simulink model "vechicle_circular_traversing"  (R2018b)
settings: Solver=FixedStepDiscrete  StartTime=0.0  StopTime=TFinal  FixedStep=Ts  RelTol=1e-3
values from neighbouring files (symbols this model uses):
  cx = 2    [Test_EKF_circular_trajectory.m]
  cy = 2    [Test_EKF_circular_trajectory.m]
  muWx = 0    [Test_EKF_circular_trajectory.m]
  muWy = 0    [Test_EKF_circular_trajectory.m]
  P0 = [1;1]    [Test_EKF_circular_trajectory.m]
  sigB = 1e-1    (= 0.1)    [Test_EKF_circular_trajectory.m]
  sigR = 1e-1    (= 0.1)    [Test_EKF_circular_trajectory.m]
  sigWx = 1e-7    (= 1e-07)    [Test_EKF_circular_trajectory.m]
  sigWy = 1e-7    (= 1e-07)    [Test_EKF_circular_trajectory.m]
  Ts = 0.01    [KF_Pendulum_parameter.m]    (also in Test_EKF_circular_trajectory.m)
  V0 = [-0.25;0.25]    [Test_EKF_circular_trajectory.m]
  wx = 0    [Test_EKF_circular_trajectory.m]
  wy = 0    [Test_EKF_circular_trajectory.m]
  Z = 2    [Test_EKF_circular_trajectory.m]
undefined symbols (not defined in the file or in its folder): randraw
settings Model: Creator=chpark  LastModifiedBy=chpark

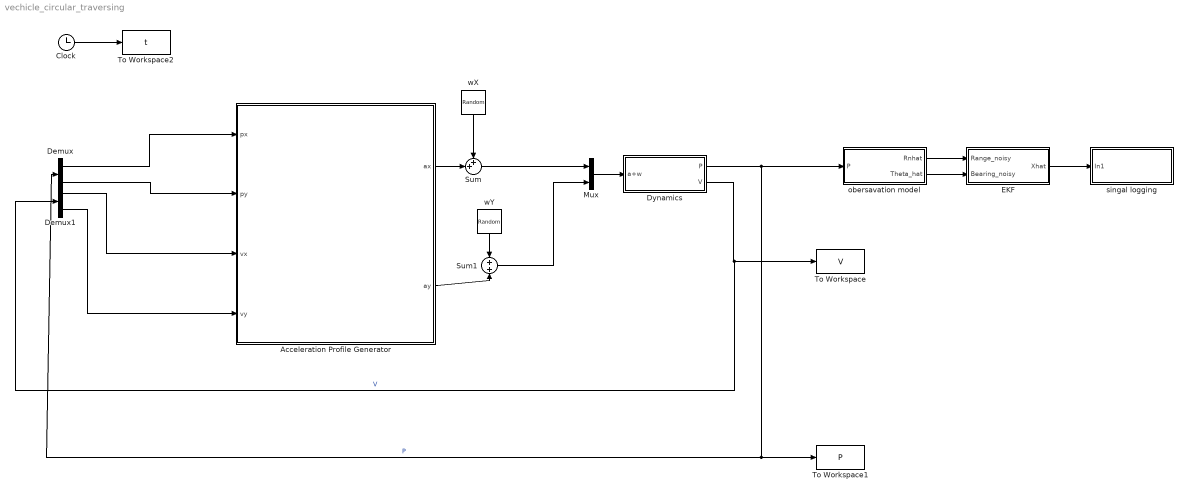
== system vechicle_circular_traversing ==
  Acceleration Profile Generator : Subsystem
  Clock : Clock
  Demux : Demux  Outputs=2
  Demux1 : Demux  Outputs=2
  Dynamics : Subsystem
  EKF : Subsystem
  Mux : Mux  Inputs=2
  Sum : Sum  Inputs=++|
  Sum1 : Sum
  To Workspace : ToWorkspace  VariableName=V  SampleTime=-1
  To Workspace1 : ToWorkspace  VariableName=P  SampleTime=-1
  To Workspace2 : ToWorkspace  VariableName=t  SampleTime=-1
  obersavation model : Subsystem
  singal logging : Subsystem
  wX : RandomNumber  Mean=muWx  Variance=sigWx  Seed=2^wx  SampleTime=Ts
  wY : RandomNumber  Mean=muWy  Variance=sigWy  Seed=2^wy  SampleTime=Ts
  wires:
  Acceleration Profile Generator/1(ax) -> Sum/2
  wX/1 -> Sum/1
  wY/1 -> Sum1/1
  Acceleration Profile Generator/2(ay) -> Sum1/2
  Sum1/1 -> Mux/2
  Sum/1 -> Mux/1
  Mux/1 -> Dynamics/1(a+w)
  Dynamics/1(P) -> obersavation model/1(P), To Workspace1/1, Demux/1  "P"
  obersavation model/1(Rnhat) -> EKF/1(Range_noisy)
  obersavation model/2(Theta_hat) -> EKF/2(Bearing_noisy)
  EKF/1(Xhat) -> singal logging/1(In1)
  Demux/1 -> Acceleration Profile Generator/1(px)
  Demux/2 -> Acceleration Profile Generator/2(py)
  Demux1/1 -> Acceleration Profile Generator/3(vx)
  Demux1/2 -> Acceleration Profile Generator/4(vy)
  Dynamics/2(V) -> Demux1/1, To Workspace/1  "V"
  Clock/1 -> To Workspace2/1

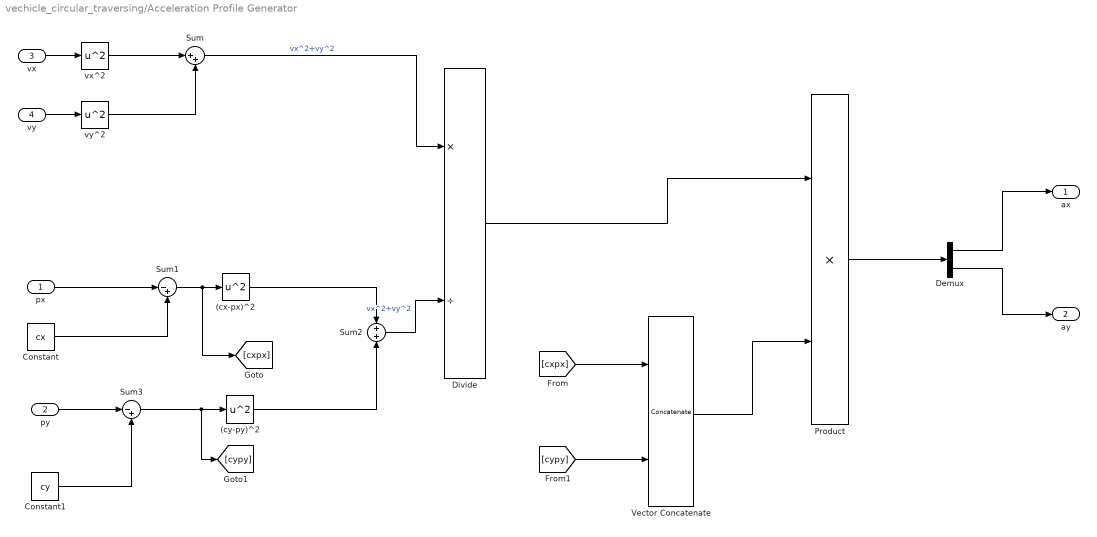
== system vechicle_circular_traversing/Acceleration Profile Generator ==
  px : Inport
  py : Inport  Port=2
  vx : Inport  Port=3
  vy : Inport  Port=4
  (cx-px)^2 : Math  Operator=square  SaturateOnIntegerOverflow=on
  (cy-py)^2 : Math  Operator=square  SaturateOnIntegerOverflow=on
  Constant : Constant  Value=cx
  Constant1 : Constant  Value=cy
  Demux : Demux  Outputs=2
  Divide : Product  Inputs=*/
  Product : Product
  Sum : Sum  Inputs=|++
  Sum1 : Sum  Inputs=|-+
  Sum2 : Sum
  Sum3 : Sum  Inputs=|-+
  Vector Concatenate : Concatenate
  vx^2 : Math  Operator=square  SaturateOnIntegerOverflow=on
  vy^2 : Math  Operator=square  SaturateOnIntegerOverflow=on
  ax : Outport
  ay : Outport  Port=2
  wires:
  Vector Concatenate/1 -> Product/2
  Divide/1 -> Product/1
  vy^2/1 -> Sum/2
  Sum/1 -> Divide/1  "vx^2+vy^2"
  vy/1 -> vy^2/1
  Demux/2 -> ay/1
  Demux/1 -> ax/1
  vx/1 -> vx^2/1
  px/1 -> Sum1/1
  Constant/1 -> Sum1/2
  Sum1/1 -> [cxpx], (cx-px)^2/1
  (cx-px)^2/1 -> Sum2/1
  [cxpx] -> Vector Concatenate/1
  Sum2/1 -> Divide/2  "vx^2+vy^2"
  Sum3/1 -> [cypy], (cy-py)^2/1
  [cypy] -> Vector Concatenate/2
  Constant1/1 -> Sum3/2
  Product/1 -> Demux/1
  py/1 -> Sum3/1
  (cy-py)^2/1 -> Sum2/2
  vx^2/1 -> Sum/1

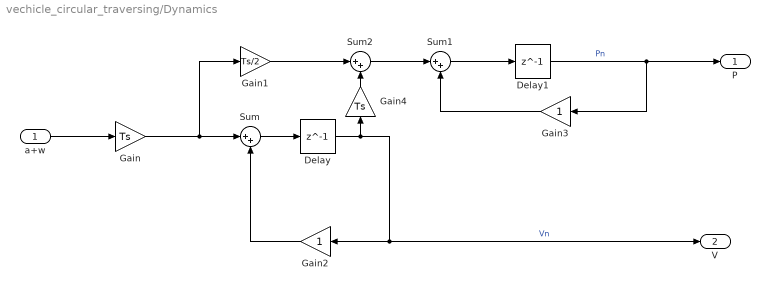
== system vechicle_circular_traversing/Dynamics ==
  a+w : Inport
  Delay : Delay  DelayLength=1  InitialCondition=V0
  Delay1 : Delay  DelayLength=1  InitialCondition=P0
  Gain : Gain  Gain=Ts
  Gain1 : Gain  Gain=Ts/2
  Gain2 : Gain
  Gain3 : Gain
  Gain4 : Gain  Gain=Ts
  Sum : Sum  Inputs=|++
  Sum1 : Sum  Inputs=|++
  Sum2 : Sum  Inputs=|++
  P : Outport
  V : Outport  Port=2
  wires:
  a+w/1 -> Gain/1
  Gain/1 -> Gain1/1, Sum/1
  Sum/1 -> Delay/1
  Gain2/1 -> Sum/2
  Gain3/1 -> Sum1/2
  Sum1/1 -> Delay1/1
  Delay1/1 -> Gain3/1, P/1  "Pn"
  Gain1/1 -> Sum2/1
  Gain4/1 -> Sum2/2
  Delay/1 -> Gain2/1, V/1, Gain4/1  "Vn"
  Sum2/1 -> Sum1/1

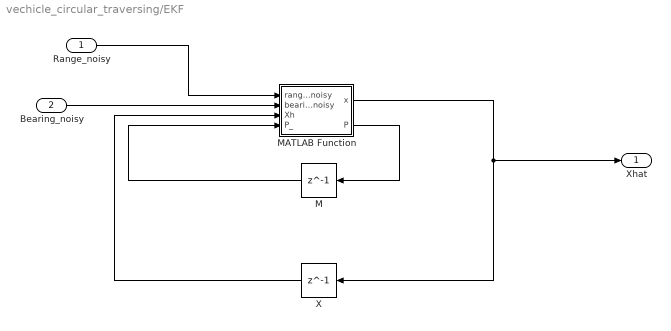
== system vechicle_circular_traversing/EKF ==
  Range_noisy : Inport
  Bearing_noisy : Inport  Port=2
  M : Delay  DelayLength=1  InitialCondition=zeros(4,4)
  MATLAB Function : MATLAB Function  TreatAsAtomicUnit=on
  X : Delay  DelayLength=1  InitialCondition=[P0;V0]
  Xhat : Outport
  wires:
  Range_noisy/1 -> MATLAB Function/1(range_noisy)
  Bearing_noisy/1 -> MATLAB Function/2(bearing_noisy)
  M/1 -> MATLAB Function/4(P_)
  MATLAB Function/2(P) -> M/1
  MATLAB Function/1(x) -> X/1, Xhat/1
  X/1 -> MATLAB Function/3(Xh)

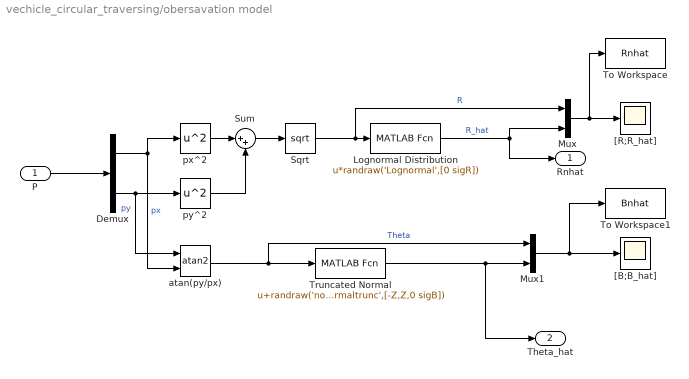
== system vechicle_circular_traversing/obersavation model ==
  P : Inport
  Demux : Demux  Outputs=2
  Lognormal Distribution : MATLABFcn  MATLABFcn=u*randraw('Lognormal',[0 sigR])
  Mux : Mux  Inputs=2
  Mux1 : Mux  Inputs=2
  Sqrt : Sqrt  SaturateOnIntegerOverflow=on
  Sum : Sum  Inputs=|++
  To Workspace : ToWorkspace  VariableName=Rnhat  SampleTime=-1
  To Workspace1 : ToWorkspace  VariableName=Bnhat  SampleTime=-1
  Truncated Normal : MATLABFcn  MATLABFcn=u+randraw('normaltrunc',[-Z,Z,0 sigB])
  "[B;B_hat]" : Scope
  "[R;R_hat]" : Scope
  atan(py/px) : Trigonometry  Operator=atan2
  px^2 : Math  Operator=square  SaturateOnIntegerOverflow=on
  py^2 : Math  Operator=square  SaturateOnIntegerOverflow=on
  Rnhat : Outport
  Theta_hat : Outport  Port=2
  wires:
  Demux/1 -> px^2/1, atan(py/px)/2  "px"
  Demux/2 -> atan(py/px)/1, py^2/1  "py"
  px^2/1 -> Sum/1
  py^2/1 -> Sum/2
  Sum/1 -> Sqrt/1
  Sqrt/1 -> Mux/1, Lognormal Distribution/1  "R"
  Lognormal Distribution/1 -> Mux/2, Rnhat/1  "R_hat"
  atan(py/px)/1 -> Truncated Normal/1, Mux1/1  "Theta"
  Truncated Normal/1 -> Theta_hat/1, Mux1/2
  Mux1/1 -> To Workspace1/1, "[B;B_hat]"/1
  Mux/1 -> To Workspace/1, "[R;R_hat]"/1
  P/1 -> Demux/1

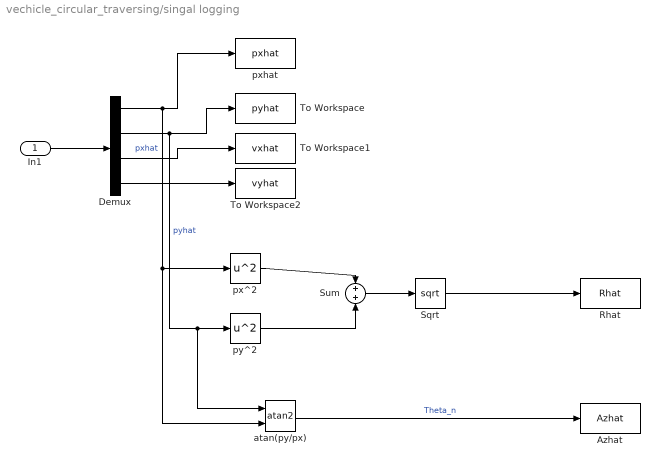
== system vechicle_circular_traversing/singal logging ==
  In1 : Inport
  Azhat : ToWorkspace  VariableName=Azhat  SampleTime=-1
  Demux : Demux
  Rhat : ToWorkspace  VariableName=Rhat  SampleTime=-1
  Sqrt : Sqrt  SaturateOnIntegerOverflow=on
  Sum : Sum
  To Workspace : ToWorkspace  VariableName=pyhat  SampleTime=-1
  To Workspace1 : ToWorkspace  VariableName=vxhat  SampleTime=-1
  To Workspace2 : ToWorkspace  VariableName=vyhat  SampleTime=-1
  atan(py/px) : Trigonometry  Operator=atan2
  px^2 : Math  Operator=square  SaturateOnIntegerOverflow=on
  pxhat : ToWorkspace  VariableName=pxhat  SampleTime=-1
  py^2 : Math  Operator=square  SaturateOnIntegerOverflow=on
  wires:
  In1/1 -> Demux/1
  Demux/2 -> To Workspace/1, atan(py/px)/1, py^2/1  "pyhat"
  Demux/3 -> To Workspace1/1
  Demux/4 -> To Workspace2/1
  Sqrt/1 -> Rhat/1
  Sum/1 -> Sqrt/1
  atan(py/px)/1 -> Azhat/1  "Theta_n"
  py^2/1 -> Sum/2
  px^2/1 -> Sum/1
  Demux/1 -> atan(py/px)/2, px^2/1, pxhat/1  "pxhat"

== matlab function vechicle_circular_traversing/EKF/MATLAB Function ==
  data: range_noisy input; x output; bearing_noisy input; Xh input; P_ input; P output
function [x,P] = EKF(range_noisy,bearing_noisy,Xh,P_)
% 샘플링 주기
Ts = 1/100;

sigWx = 1e-7;
sigWy = 1e-7;

sigR = 1e-1;
sigB = 1e-1;

Q = [sigWx 0;0 sigWy];
R = [sigB 0;0 sigB];
% 원의 중심점
cx = 2;
cy = 2;

px = Xh(1);
py = Xh(2);
vx = Xh(3);
vy = Xh(4);
% 자코비안 변환
A= Ajacob(cx,cy,px,py,vx,vy,Ts);
L = Lmat(Ts);

Pos = [px;py];
Vel = [vx;vy];

ax = ((vx^2 + vy^2)*(cx - px))/((cx-px)^2 + (cy-py)^2);
ay = ((vx^2 + vy^2)*(cy - py))/((cx-px)^2 + (cy-py)^2);

alph = [ax;ay];
% 추정값과 오차 공분산 예측
xp = [Pos;zeros(2,1)] + [Ts*Vel;Vel] + Ts*[zeros(2,1);alph] + ((Ts^2)/2)*[alph;zeros(2,1)];
Pp = A*P_*A' + L*Q*L';

pxup = xp(1);
pyup = xp(2);
vxup = xp(3);
vyup = xp(4);
% 자코비안 변환
H = Hjacob(pxup,pyup);
M = Mjacob(pxup,pyup);
% 칼만 이득 계산
K = Pp*H'*inv(H*Pp*H' + M*R*M');
% 추정값 계산
x = xp + K*([range_noisy;bearing_noisy] - [(xp(1)^2 + xp(2)^2) ^0.5;atan2(xp(2),xp(1))]);
% 오차 공분산 계산
P = (eye(4) - K*H)*Pp;
end

function A = Ajacob(cx,cy,px,py,vx,vy,Ts)
a = (cx-px)^2 + (cy-py)^2;
b = vx^2 + vy^2;
c= b/a;

a11 = 1+c*((cx-px)^2/a - (1/2))*Ts^2;
a12 = c*(1/a)*(cx-px)*(cy-py)*Ts^2;
a13 = (1/a)*vx*(cx-px)*Ts^2;
a14 = (1/a)*vy*(cy-py)*Ts^2;

a21 = c*(1/a)*(cx-px)*(cy-py)*Ts^2;
a22 = 1+(Ts^2*c*((1/a)*(cy-py)^2 - (1/2)));
a23 = (Ts/a)*(vx*(cy-py));
a24 =Ts + ((vy/a)*(cy-py))*Ts^2;

a31 = c*(Ts*(2/a)*(cx-px)^2-Ts);
a32 = (2*Ts*c)*(1/a)*(cy-py)*(cx-px);
a33 = 1+(2*Ts/a)*vx*(cx-px);
a34 = (2*Ts/a)*vy*(cx-px);

a41 = 2*(c/a)*(cx-px)*(cy-py);
a42 = c*((2/a)*(cy-py)^2 - 1)*Ts;
a43 = (2*Ts/a)*vx*(cy-py);
a44 = 1+(2*Ts/a)*(cy-py);

A = [a11 a12 a13 a14;
     a21 a22 a23 a24;
     a31 a32 a33 a34;
     a41 a42 a43 a44];
end

function L = Lmat(Ts)

l11 = (Ts^2)/2;
l12 =0;
l21 =0;
l22 =l11;
l31 =Ts;
l32 =0;
l41 =0;
l42 =Ts;

L = [l11 l12; l21 l22; l31 l32; l41 l42];
end

function H = Hjacob(pxup,pyup)

H = [0 0 0 0; -pyup/(pxup^2 + pyup^2) , pxup/(pxup^2 + pyup^2), 0, 0];
end

function M = Mjacob(pxup,pyup)

M = [(pxup^2 + pyup^2)^(1/2),0 ; 0,1];
end
